simulink model "Controlador_codigo_export"  (R2023b)
settings: Solver=FixedStepAuto  StartTime=0.0  StopTime=20  FixedStep=0.00006  RelTol=1e-3
undefined symbols (not defined in the file): alpha_cu, b_eq, C_ts, g, J_eq, k_l, L_d, L_ls, L_q, lambda_m, magnitude, P_p, r, R_sREF, R_ts_amb, T_amb, T_ld, T_sdis, T_sREF, Tau_sens_temp, Vsat, w_n_modulador, w_n_sens_corr, w_n_sens_pos, zeta_mod, zeta_sens
libraries: SignalEditorBlockLib x2
settings Model: Creator=tomas  LastModifiedBy=tomas

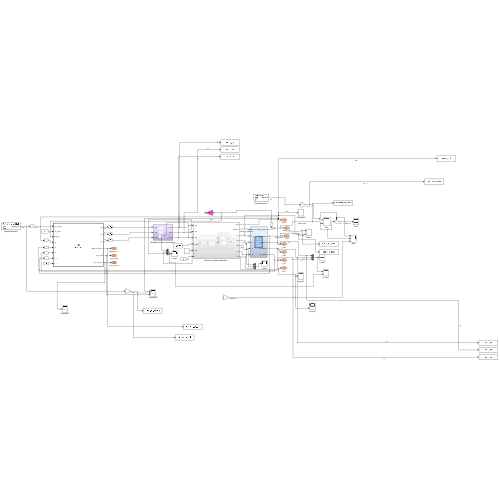
[thumbnail: Simulink's stored preview of the top-level diagram]
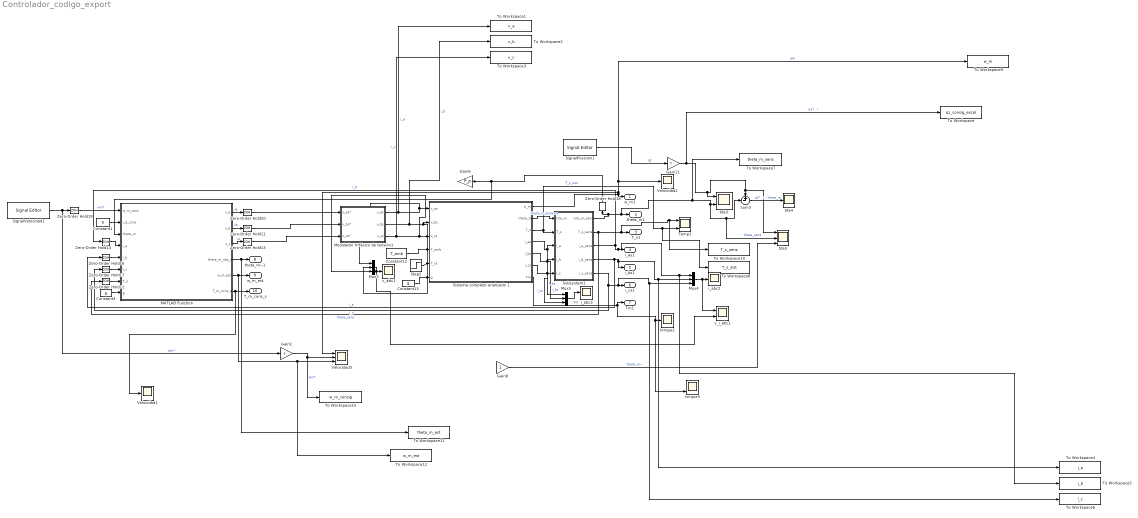
== system Controlador_codigo_export ==
  Constant1 : Constant  Value=0
  Constant12 : Constant  Value=T_amb
  Constant13 : Constant  Value=g
  Constant3 : Constant  Value=g
  Gain1 : Gain  Gain=r
  Gain11 : Gain  Gain=r
  Gain6 : Gain  Gain=P_p
  Gain8 : Gain
  MATLAB Function : MATLAB Function  TreatAsAtomicUnit=on
  Modulador trifásico de tensión1 : Subsystem
  Mux3 : Mux  Inputs=3
  Mux4 : Mux  Inputs=3
  Mux5 : Mux  Inputs=3
  SignalPosicion1 : SignalEditorBlockLib/Signal Editor  FileName=D:\Facu\Final AyME\Final-AyME\Simulink_LC\Simulacion\Signal\Perfil_trap_q1.mat  ActiveScenario=Scenarioq1  ActiveSignal=Signalq1  IsBus=off  OutputBusObjectStr=Bus: BusObject  SampleTime=0  ZeroCross=off  OutputAfterFinalValue=Holding final value  Unit=inherit  PreserveSignalName=on  ApplySigPropsToAllScenarios=on  ApplySigPropsToAllSignals=off
  SignalVelocidad1 : SignalEditorBlockLib/Signal Editor  FileName=D:\Facu\Final AyME\Final-AyME\Simulink_LC\Simulacion\Signal\Perfil_trap_velocidad.mat  ActiveScenario=Scenario_velocidad  ActiveSignal=Signal_vel  IsBus=off  OutputBusObjectStr=Bus: BusObject  SampleTime=0  ZeroCross=off  OutputAfterFinalValue=Holding final value  Unit=inherit  PreserveSignalName=on  ApplySigPropsToAllScenarios=on  ApplySigPropsToAllSignals=off
  Sistema completo analizado 1 : Subsystem
  Step2 : Step  Time=7.5  After=T_ld*0  SampleTime=0
  Subsystem1 : Subsystem
  Sum3 : Sum  Inputs=+-|
  Temp1 : Scope  NumInputPorts=2
  To Workspace : ToWorkspace  VariableName=q1_consig_escal  SaveFormat=Structure With Time  SampleTime=-1
  To Workspace1 : ToWorkspace  VariableName=v_a  SaveFormat=Structure With Time  SampleTime=-1
  To Workspace10 : ToWorkspace  VariableName=T_s_sens  SaveFormat=Structure With Time  SampleTime=-1
  To Workspace11 : ToWorkspace  VariableName=theta_m_est  SaveFormat=Structure With Time  SampleTime=-1
  To Workspace12 : ToWorkspace  VariableName=w_m_est  SaveFormat=Structure With Time  SampleTime=-1
  To Workspace15 : ToWorkspace  VariableName=w_m_consig  SaveFormat=Structure With Time  SampleTime=-1
  To Workspace2 : ToWorkspace  VariableName=v_b  SaveFormat=Structure With Time  SampleTime=-1
  To Workspace3 : ToWorkspace  VariableName=v_c  SaveFormat=Structure With Time  SampleTime=-1
  To Workspace4 : ToWorkspace  VariableName=i_a  SaveFormat=Structure With Time  SampleTime=-1
  To Workspace5 : ToWorkspace  VariableName=i_b  SaveFormat=Structure With Time  SampleTime=-1
  To Workspace6 : ToWorkspace  VariableName=i_c  SaveFormat=Structure With Time  SampleTime=-1
  To Workspace7 : ToWorkspace  VariableName=theta_m_sens  SaveFormat=Structure With Time  SampleTime=-1
  To Workspace8 : ToWorkspace  VariableName=T_s_sist  SaveFormat=Structure With Time  SampleTime=-1
  To Workspace9 : ToWorkspace  VariableName=w_m  SaveFormat=Structure With Time  SampleTime=-1
  Velocidad1 : Scope
  Velocidad2 : Scope
  Velocidad3 : Scope  NumInputPorts=3
  Zero-Order Hold{11..14,16..20} (9 alike) : ZeroOrderHold  SampleTime=T_sdis
  i_abc2 : Scope
  i_abc3 : Scope
  tita3 : Scope  NumInputPorts=2
  tita4 : Scope
  tita5 : Scope  NumInputPorts=3
  torque2 : Scope
  torque3 : Scope  NumInputPorts=2
  v_abc1 : Scope
  v_i_abc1 : Scope  NumInputPorts=2
  w_m1 : Outport
  theta_m1 : Outport  Port=2
  T_s1 : Outport  Port=3
  i_as1 : Outport  Port=4
  i_bs1 : Outport  Port=5
  i_cs1 : Outport  Port=6
  Tm1 : Outport  Port=7
  theta_m~1 : Outport  Port=8
  w_m_est : Outport  Port=9
  T_m_cons_s : Outport  Port=10
  wires:
  Sistema completo analizado 1/7(Tm) -> torque3/2, torque2/1, Tm1/1  "Tm"
  Zero-Order Hold11/1 -> Modulador trifásico de tensión1/2(v_bs*)
  Zero-Order Hold16/1 -> MATLAB Function/5(i_b)
  Zero-Order Hold18/1 -> MATLAB Function/3(theta_m), Gain6/1
  Step2/1 -> Sistema completo analizado 1/5(T_ld)
  MATLAB Function/2(v_b) -> Zero-Order Hold11/1  "vb"
  Sistema completo analizado 1/5(i_bs) -> Subsystem1/4(i_b), Mux5/2  "i_bs"
  Zero-Order Hold17/1 -> MATLAB Function/6(i_c)
  Zero-Order Hold13/1 -> Modulador trifásico de tensión1/3(v_cs*)
  Sistema completo analizado 1/2(theta_m) -> Subsystem1/1(tita_m)  "theta_m_sistema"
  Zero-Order Hold20/1 -> Modulador trifásico de tensión1/1(v_as*)
  Zero-Order Hold14/1 -> MATLAB Function/4(i_a)
  MATLAB Function/1(v_a) -> Zero-Order Hold20/1  "va"
  Mux4/1 -> v_i_abc1/1, i_abc2/1
  Constant1/1 -> MATLAB Function/2(i_d_cons)
  Mux5/1 -> i_abc3/1
  Sistema completo analizado 1/4(i_as) -> Subsystem1/3(i_a), Mux5/1  "i_as"
  Gain8/1 -> tita5/3  "theta_m~"
  Sum3/1 -> tita4/1  "q1* . r - theta_m"
  Constant3/1 -> MATLAB Function/8(g)
  Mux3/1 -> v_i_abc1/2, v_abc1/1
  Constant13/1 -> Sistema completo analizado 1/6(g)
  MATLAB Function/3(v_c) -> Zero-Order Hold13/1  "vc"
  Sistema completo analizado 1/3(T_s) -> Subsystem1/2(T_s), To Workspace8/1, Temp1/2  "T_s_sist"
  Sistema completo analizado 1/6(i_cs) -> Subsystem1/5(i_c), Mux5/3  "i_cs"
  Subsystem1/1(tita_m_sens) -> Zero-Order Hold18/1, To Workspace7/1, tita5/2, Sum3/2, tita3/2, theta_m1/1  "theta_sens"
  Constant12/1 -> Sistema completo analizado 1/4(T_amb)
  Zero-Order Hold12/1 -> MATLAB Function/7(T_s)
  MATLAB Function/6(T_m_cons_s) -> Velocidad1/1, T_m_cons_s/1
  Zero-Order Hold19/1 -> MATLAB Function/1(w_m_cons)  "wm*"
  SignalPosicion1/1 -> Gain11/1  "q1"
  Gain1/1 -> To Workspace15/1, Velocidad3/2  "wm*"
  Subsystem1/5(i_c_sens) -> Zero-Order Hold17/1, To Workspace6/1, Mux4/3, i_cs1/1  "i_c"
  Subsystem1/4(i_b_sens) -> i_bs1/1, To Workspace4/1, Mux4/2, Zero-Order Hold16/1  "i_a"
  Subsystem1/3(i_a_sens) -> To Workspace5/1, Mux4/1, i_as1/1, Zero-Order Hold14/1  "i_b"
  Subsystem1/2(T_s_sens) -> Zero-Order Hold12/1, To Workspace10/1, Temp1/1, T_s1/1  "theta_sens"
  Gain11/1 -> To Workspace/1, tita3/1, tita5/1, Sum3/1  "q1* . r"
  Sistema completo analizado 1/1(w_m) -> To Workspace9/1, Velocidad2/1, Velocidad3/1, w_m1/1  "wm"
  Modulador trifásico de tensión1/2(v_bs) -> To Workspace2/1, Mux3/2, Sistema completo analizado 1/2(v_bs)  "i_b"
  Modulador trifásico de tensión1/3(v_cs) -> To Workspace3/1, Mux3/3, Sistema completo analizado 1/3(v_cs)  "i_c"
  Modulador trifásico de tensión1/1(v_as) -> To Workspace1/1, Mux3/1, Sistema completo analizado 1/1(v_as)  "i_a"
  SignalVelocidad1/1 -> Gain1/1, Zero-Order Hold19/1  "wm*"
  MATLAB Function/5(w_m_est) -> To Workspace12/1, Velocidad3/3, w_m_est/1
  MATLAB Function/4(theta_m_obs_s) -> To Workspace11/1, theta_m~1/1

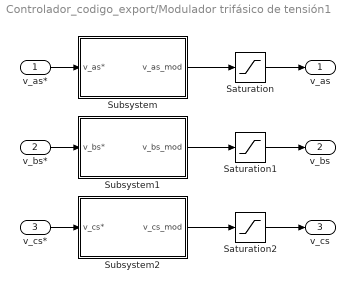
== system Controlador_codigo_export/Modulador trifásico de tensión1 ==
  v_as* : Inport
  v_bs* : Inport  Port=2
  v_cs* : Inport  Port=3
  Saturation : Saturate  UpperLimit=Vsat  LowerLimit=-Vsat
  Saturation1 : Saturate  UpperLimit=Vsat  LowerLimit=-Vsat
  Saturation2 : Saturate  UpperLimit=Vsat  LowerLimit=-Vsat
  Subsystem : Subsystem
  Subsystem1 : Subsystem
  Subsystem2 : Subsystem
  v_as : Outport
  v_bs : Outport  Port=2
  v_cs : Outport  Port=3
  wires:
  Subsystem/1(v_as_mod) -> Saturation/1
  Subsystem1/1(v_bs_mod) -> Saturation1/1
  Subsystem2/1(v_cs_mod) -> Saturation2/1
  v_cs*/1 -> Subsystem2/1(v_cs*)
  v_bs*/1 -> Subsystem1/1(v_bs*)
  v_as*/1 -> Subsystem/1(v_as*)
  Saturation/1 -> v_as/1
  Saturation1/1 -> v_bs/1
  Saturation2/1 -> v_cs/1

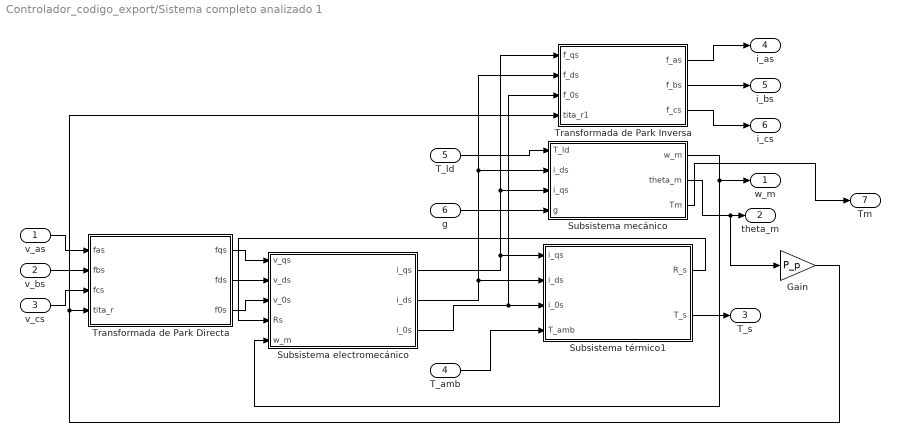
== system Controlador_codigo_export/Sistema completo analizado 1 ==
  v_as : Inport
  v_bs : Inport  Port=2
  v_cs : Inport  Port=3
  T_amb : Inport  Port=4
  T_ld : Inport  Port=5
  g : Inport  Port=6
  Gain : Gain  Gain=P_p
  Subsistema electromecánico : Subsystem
  Subsistema mecánico : Subsystem
  Subsistema térmico1 : Subsystem
  Transformada de Park Directa : Subsystem
  Transformada de Park Inversa : Subsystem
  w_m : Outport
  theta_m : Outport  Port=2
  T_s : Outport  Port=3
  i_as : Outport  Port=4
  i_bs : Outport  Port=5
  i_cs : Outport  Port=6
  Tm : Outport  Port=7
  wires:
  Transformada de Park Inversa/3(f_cs) -> i_cs/1
  Subsistema mecánico/1(w_m) -> w_m/1, Subsistema electromecánico/5(w_m)
  Subsistema electromecánico/3(i_0s) -> Subsistema térmico1/3(i_0s), Transformada de Park Inversa/3(f_0s)
  Transformada de Park Directa/1(fqs) -> Subsistema electromecánico/1(v_qs)
  Subsistema térmico1/2(T_s) -> T_s/1
  Transformada de Park Directa/3(f0s) -> Subsistema electromecánico/3(v_0s)
  Subsistema electromecánico/2(i_ds) -> Subsistema térmico1/2(i_ds), Transformada de Park Inversa/2(f_ds), Subsistema mecánico/2(i_ds)
  Gain/1 -> Transformada de Park Inversa/4(tita_r1), Transformada de Park Directa/4(tita_r)
  T_ld/1 -> Subsistema mecánico/1(T_ld)
  Transformada de Park Directa/2(fds) -> Subsistema electromecánico/2(v_ds)
  Transformada de Park Inversa/2(f_bs) -> i_bs/1
  v_bs/1 -> Transformada de Park Directa/2(fbs)
  T_amb/1 -> Subsistema térmico1/4(T_amb)
  Transformada de Park Inversa/1(f_as) -> i_as/1
  v_as/1 -> Transformada de Park Directa/1(fas)
  Subsistema mecánico/2(theta_m) -> Gain/1, theta_m/1
  v_cs/1 -> Transformada de Park Directa/3(fcs)
  Subsistema electromecánico/1(i_qs) -> Transformada de Park Inversa/1(f_qs), Subsistema mecánico/3(i_qs), Subsistema térmico1/1(i_qs)
  Subsistema térmico1/1(R_s) -> Subsistema electromecánico/4(Rs)
  g/1 -> Subsistema mecánico/4(g)
  Subsistema mecánico/3(Tm) -> Tm/1

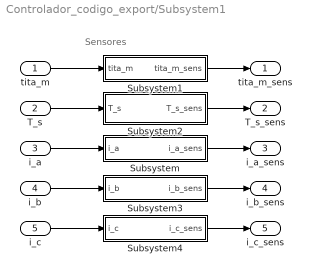
== system Controlador_codigo_export/Subsystem1 ==
  note: Sensores
  tita_m : Inport
  T_s : Inport  Port=2
  i_a : Inport  Port=3
  i_b : Inport  Port=4
  i_c : Inport  Port=5
  Subsystem : Subsystem
  Subsystem1 : Subsystem
  Subsystem2 : Subsystem
  Subsystem3 : Subsystem
  Subsystem4 : Subsystem
  tita_m_sens : Outport
  T_s_sens : Outport  Port=2
  i_a_sens : Outport  Port=3
  i_b_sens : Outport  Port=4
  i_c_sens : Outport  Port=5
  wires:
  tita_m/1 -> Subsystem1/1(tita_m)
  T_s/1 -> Subsystem2/1(T_s)
  i_a/1 -> Subsystem/1(i_a)
  i_b/1 -> Subsystem3/1(i_b)
  i_c/1 -> Subsystem4/1(i_c)
  Subsystem1/1(tita_m_sens) -> tita_m_sens/1
  Subsystem2/1(T_s_sens) -> T_s_sens/1
  Subsystem/1(i_a_sens) -> i_a_sens/1
  Subsystem3/1(i_b_sens) -> i_b_sens/1
  Subsystem4/1(i_c_sens) -> i_c_sens/1

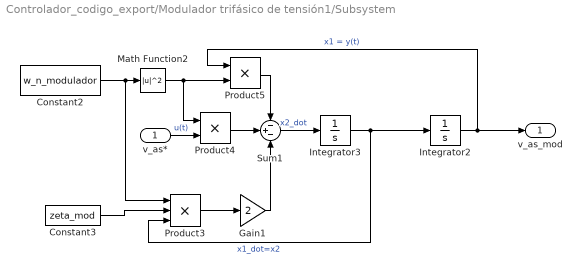
== system Controlador_codigo_export/Modulador trifásico de tensión1/Subsystem ==
  v_as* : Inport
  Constant2 : Constant  Value=w_n_modulador
  Constant3 : Constant  Value=zeta_mod
  Gain1 : Gain  Gain=2
  Integrator2 : Integrator
  Integrator3 : Integrator
  Math Function2 : Math  Operator=magnitude^2
  Product3 : Product  Inputs=3
  Product4 : Product
  Product5 : Product
  Sum1 : Sum  Inputs=-+-
  v_as_mod : Outport
  wires:
  Math Function2/1 -> Product5/2, Product4/1
  Integrator3/1 -> Product3/3, Integrator2/1  "x1_dot=x2"
  v_as*/1 -> Product4/2  "u(t)"
  Product4/1 -> Sum1/2
  Sum1/1 -> Integrator3/1  "x2_dot"
  Integrator2/1 -> v_as_mod/1, Product5/1  "x1 = y(t)"
  Gain1/1 -> Sum1/3
  Product3/1 -> Gain1/1
  Constant2/1 -> Product3/1, Math Function2/1
  Product5/1 -> Sum1/1
  Constant3/1 -> Product3/2

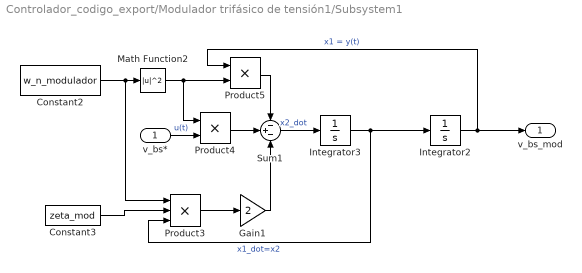
== system Controlador_codigo_export/Modulador trifásico de tensión1/Subsystem1 ==
  v_bs* : Inport
  Constant2 : Constant  Value=w_n_modulador
  Constant3 : Constant  Value=zeta_mod
  Gain1 : Gain  Gain=2
  Integrator2 : Integrator
  Integrator3 : Integrator
  Math Function2 : Math  Operator=magnitude^2
  Product3 : Product  Inputs=3
  Product4 : Product
  Product5 : Product
  Sum1 : Sum  Inputs=-+-
  v_bs_mod : Outport
  wires:
  Math Function2/1 -> Product5/2, Product4/1
  Integrator3/1 -> Product3/3, Integrator2/1  "x1_dot=x2"
  v_bs*/1 -> Product4/2  "u(t)"
  Product4/1 -> Sum1/2
  Sum1/1 -> Integrator3/1  "x2_dot"
  Integrator2/1 -> v_bs_mod/1, Product5/1  "x1 = y(t)"
  Gain1/1 -> Sum1/3
  Product3/1 -> Gain1/1
  Constant2/1 -> Product3/1, Math Function2/1
  Product5/1 -> Sum1/1
  Constant3/1 -> Product3/2

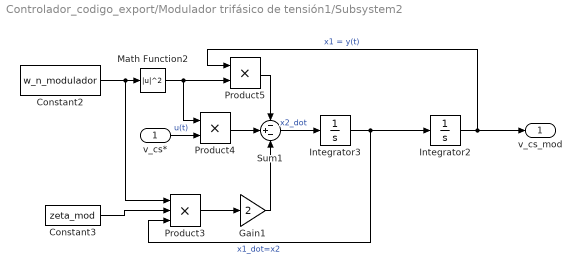
== system Controlador_codigo_export/Modulador trifásico de tensión1/Subsystem2 ==
  v_cs* : Inport
  Constant2 : Constant  Value=w_n_modulador
  Constant3 : Constant  Value=zeta_mod
  Gain1 : Gain  Gain=2
  Integrator2 : Integrator
  Integrator3 : Integrator
  Math Function2 : Math  Operator=magnitude^2
  Product3 : Product  Inputs=3
  Product4 : Product
  Product5 : Product
  Sum1 : Sum  Inputs=-+-
  v_cs_mod : Outport
  wires:
  Math Function2/1 -> Product5/2, Product4/1
  Integrator3/1 -> Product3/3, Integrator2/1  "x1_dot=x2"
  v_cs*/1 -> Product4/2  "u(t)"
  Product4/1 -> Sum1/2
  Sum1/1 -> Integrator3/1  "x2_dot"
  Integrator2/1 -> v_cs_mod/1, Product5/1  "x1 = y(t)"
  Gain1/1 -> Sum1/3
  Product3/1 -> Gain1/1
  Constant2/1 -> Product3/1, Math Function2/1
  Product5/1 -> Sum1/1
  Constant3/1 -> Product3/2

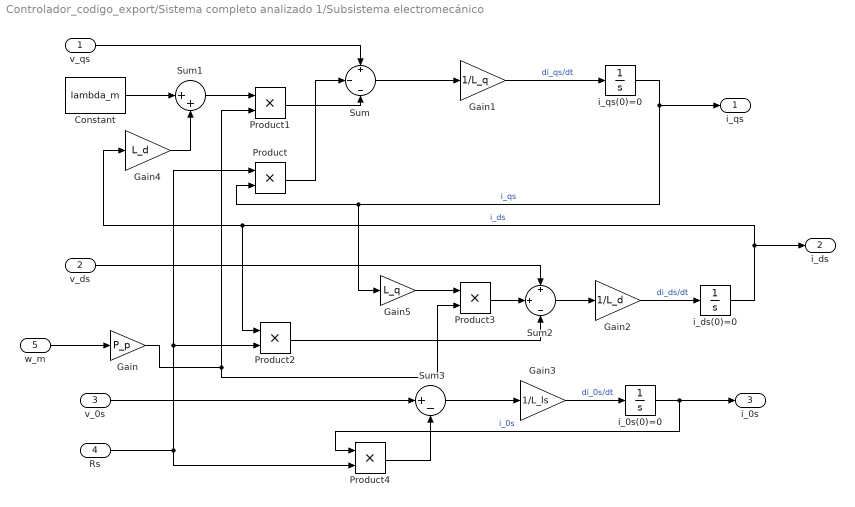
== system Controlador_codigo_export/Sistema completo analizado 1/Subsistema electromecánico ==
  v_qs : Inport
  v_ds : Inport  Port=2
  v_0s : Inport  Port=3
  Rs : Inport  Port=4
  w_m : Inport  Port=5
  Constant : Constant  Value=lambda_m
  Gain : Gain  Gain=P_p
  Gain1 : Gain  Gain=1/L_q
  Gain2 : Gain  Gain=1/L_d
  Gain3 : Gain  Gain=1/L_ls
  Gain4 : Gain  Gain=L_d
  Gain5 : Gain  Gain=L_q
  Product{,1..4} (5 alike) : Product
  Sum : Sum  Inputs=+|-|-
  Sum1 : Sum  Inputs=|++
  Sum2 : Sum  Inputs=+|+|-
  Sum3 : Sum  Inputs=|+-
  i_0s(0)=0 : Integrator
  i_ds(0)=0 : Integrator
  i_qs(0)=0 : Integrator
  i_qs : Outport
  i_ds : Outport  Port=2
  i_0s : Outport  Port=3
  wires:
  Gain1/1 -> i_qs(0)=0/1  "di_qs/dt"
  Rs/1 -> Product2/2, Product/1, Product4/2
  i_qs(0)=0/1 -> Gain5/1, Product/2, i_qs/1  "i_qs"
  Sum2/1 -> Gain2/1
  Product1/1 -> Sum/3
  Product4/1 -> Sum3/2
  v_0s/1 -> Sum3/1
  Product3/1 -> Sum2/2
  Gain3/1 -> i_0s(0)=0/1  "di_0s/dt"
  Gain/1 -> Product3/2, Product1/2
  v_qs/1 -> Sum/1
  Sum1/1 -> Product1/1
  Gain5/1 -> Product3/1
  Sum3/1 -> Gain3/1
  i_0s(0)=0/1 -> Product4/1, i_0s/1  "i_0s"
  Product2/1 -> Sum2/3
  Gain2/1 -> i_ds(0)=0/1  "di_ds/dt"
  Constant/1 -> Sum1/1
  Gain4/1 -> Sum1/2
  Sum/1 -> Gain1/1
  Product/1 -> Sum/2
  w_m/1 -> Gain/1
  i_ds(0)=0/1 -> Product2/1, Gain4/1, i_ds/1  "i_ds"
  v_ds/1 -> Sum2/1

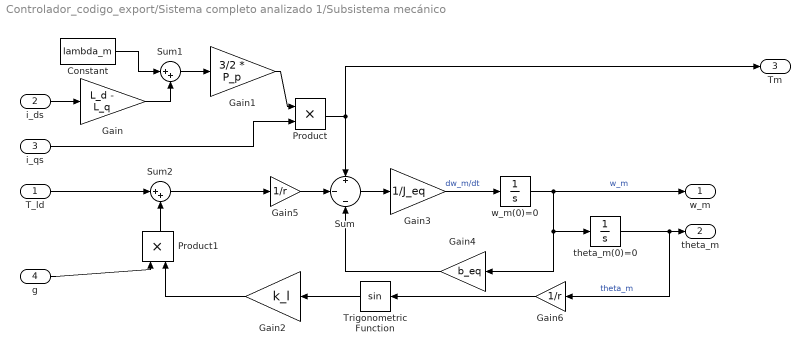
== system Controlador_codigo_export/Sistema completo analizado 1/Subsistema mecánico ==
  T_ld : Inport
  i_ds : Inport  Port=2
  i_qs : Inport  Port=3
  g : Inport  Port=4
  Constant : Constant  Value=lambda_m
  Gain : Gain  Gain=L_d - L_q
  Gain1 : Gain  Gain=3/2 * P_p
  Gain2 : Gain  Gain=k_l
  Gain3 : Gain  Gain=1/J_eq
  Gain4 : Gain  Gain=b_eq
  Gain5 : Gain  Gain=1/r
  Gain6 : Gain  Gain=1/r
  Product : Product
  Product1 : Product
  Sum : Sum  Inputs=+|-|-
  Sum1 : Sum  Inputs=|++
  Sum2 : Sum  Inputs=|++
  Trigonometric Function : Trigonometry
  theta_m(0)=0 : Integrator
  w_m(0)=0 : Integrator
  w_m : Outport
  theta_m : Outport  Port=2
  Tm : Outport  Port=3
  wires:
  w_m(0)=0/1 -> w_m/1, theta_m(0)=0/1, Gain4/1  "w_m"
  Sum/1 -> Gain3/1
  Gain3/1 -> w_m(0)=0/1  "dw_m/dt"
  i_ds/1 -> Gain/1
  Constant/1 -> Sum1/1
  Gain/1 -> Sum1/2
  Sum1/1 -> Gain1/1
  Gain1/1 -> Product/1
  i_qs/1 -> Product/2
  Gain4/1 -> Sum/3
  Gain5/1 -> Sum/2
  Trigonometric Function/1 -> Gain2/1
  Gain2/1 -> Product1/2
  theta_m(0)=0/1 -> Gain6/1, theta_m/1  "theta_m"
  T_ld/1 -> Sum2/1
  Sum2/1 -> Gain5/1
  Gain6/1 -> Trigonometric Function/1
  g/1 -> Product1/1
  Product1/1 -> Sum2/2
  Product/1 -> Sum/1, Tm/1

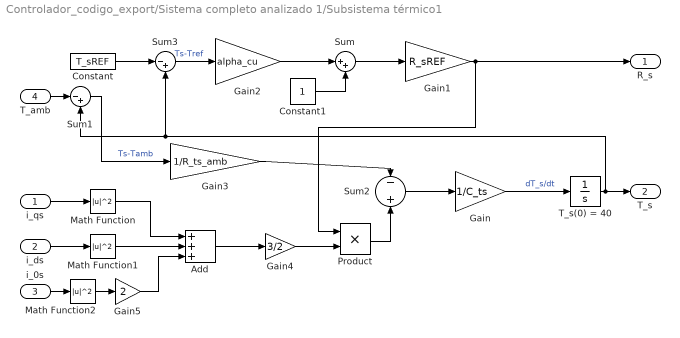
== system Controlador_codigo_export/Sistema completo analizado 1/Subsistema térmico1 ==
  i_qs : Inport
  i_ds : Inport  Port=2
  i_0s : Inport  Port=3
  T_amb : Inport  Port=4
  Add : Sum  Inputs=+++
  Constant : Constant  Value=T_sREF
  Constant1 : Constant
  Gain : Gain  Gain=1/C_ts
  Gain1 : Gain  Gain=R_sREF
  Gain2 : Gain  Gain=alpha_cu
  Gain3 : Gain  Gain=1/R_ts_amb
  Gain4 : Gain  Gain=3/2
  Gain5 : Gain  Gain=2
  Math Function : Math  Operator=magnitude^2
  Math Function1 : Math  Operator=magnitude^2
  Math Function2 : Math  Operator=magnitude^2
  Product : Product
  Sum : Sum  Inputs=|++
  Sum1 : Sum  Inputs=|-+
  Sum2 : Sum  Inputs=-|+
  Sum3 : Sum  Inputs=|-+
  T_s(0) = 40 : Integrator  InitialCondition=40
  R_s : Outport
  T_s : Outport  Port=2
  wires:
  Math Function2/1 -> Gain5/1
  Math Function/1 -> Add/1
  T_amb/1 -> Sum1/1
  Sum2/1 -> Gain/1
  Sum/1 -> Gain1/1
  Gain2/1 -> Sum/1
  Gain1/1 -> Product/1, R_s/1
  i_ds/1 -> Math Function1/1
  Gain/1 -> T_s(0) = 40/1  "dT_s/dt"
  Constant1/1 -> Sum/2
  Gain4/1 -> Product/2
  T_s(0) = 40/1 -> T_s/1, Sum3/2, Sum1/2
  Math Function1/1 -> Add/2
  i_0s/1 -> Math Function2/1
  Sum1/1 -> Gain3/1  "Ts-Tamb"
  Add/1 -> Gain4/1
  Gain5/1 -> Add/3
  i_qs/1 -> Math Function/1
  Gain3/1 -> Sum2/1
  Product/1 -> Sum2/2
  Constant/1 -> Sum3/1
  Sum3/1 -> Gain2/1  "Ts-Tref"

== system Controlador_codigo_export/Sistema completo analizado 1/Transformada de Park Directa ==
  fas : Inport
  fbs : Inport  Port=2
  fcs : Inport  Port=3
  tita_r : Inport  Port=4
  MATLAB Function1 : MATLAB Function  TreatAsAtomicUnit=on
  fqs : Outport
  fds : Outport  Port=2
  f0s : Outport  Port=3
  wires:
  fas/1 -> MATLAB Function1/1(f_as)
  MATLAB Function1/3(f_0s) -> f0s/1
  MATLAB Function1/2(f_ds) -> fds/1
  fbs/1 -> MATLAB Function1/2(f_bs)
  fcs/1 -> MATLAB Function1/3(f_cs)
  tita_r/1 -> MATLAB Function1/4(tita_r)
  MATLAB Function1/1(f_qs) -> fqs/1

== system Controlador_codigo_export/Sistema completo analizado 1/Transformada de Park Inversa ==
  f_qs : Inport
  f_ds : Inport  Port=2
  f_0s : Inport  Port=3
  tita_r1 : Inport  Port=4
  MATLAB Function2 : MATLAB Function  TreatAsAtomicUnit=on
  f_as : Outport
  f_bs : Outport  Port=2
  f_cs : Outport  Port=3
  wires:
  tita_r1/1 -> MATLAB Function2/4(tita_r)
  MATLAB Function2/2(f_bs) -> f_bs/1
  MATLAB Function2/1(f_as) -> f_as/1
  f_ds/1 -> MATLAB Function2/2(f_ds)
  MATLAB Function2/3(f_cs) -> f_cs/1
  f_0s/1 -> MATLAB Function2/3(f_0s)
  f_qs/1 -> MATLAB Function2/1(f_qs)

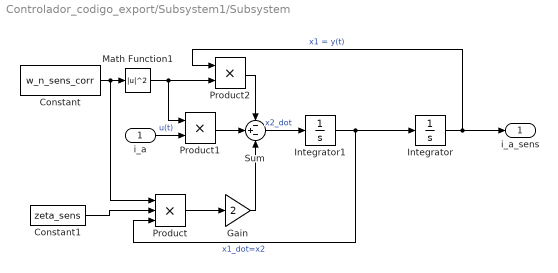
== system Controlador_codigo_export/Subsystem1/Subsystem ==
  i_a : Inport
  Constant : Constant  Value=w_n_sens_corr
  Constant1 : Constant  Value=zeta_sens
  Gain : Gain  Gain=2
  Integrator : Integrator
  Integrator1 : Integrator
  Math Function1 : Math  Operator=magnitude^2
  Product : Product  Inputs=3
  Product1 : Product
  Product2 : Product
  Sum : Sum  Inputs=-+-
  i_a_sens : Outport
  wires:
  Product1/1 -> Sum/2
  Gain/1 -> Sum/3
  Constant/1 -> Product/1, Math Function1/1
  i_a/1 -> Product1/2  "u(t)"
  Product/1 -> Gain/1
  Product2/1 -> Sum/1
  Math Function1/1 -> Product2/2, Product1/1
  Sum/1 -> Integrator1/1  "x2_dot"
  Constant1/1 -> Product/2
  Integrator1/1 -> Product/3, Integrator/1  "x1_dot=x2"
  Integrator/1 -> i_a_sens/1, Product2/1  "x1 = y(t)"

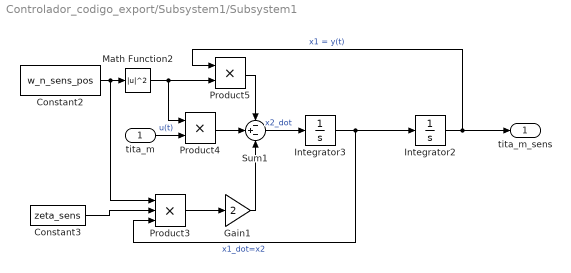
== system Controlador_codigo_export/Subsystem1/Subsystem1 ==
  tita_m : Inport
  Constant2 : Constant  Value=w_n_sens_pos
  Constant3 : Constant  Value=zeta_sens
  Gain1 : Gain  Gain=2
  Integrator2 : Integrator
  Integrator3 : Integrator
  Math Function2 : Math  Operator=magnitude^2
  Product3 : Product  Inputs=3
  Product4 : Product
  Product5 : Product
  Sum1 : Sum  Inputs=-+-
  tita_m_sens : Outport
  wires:
  Constant2/1 -> Product3/1, Math Function2/1
  Gain1/1 -> Sum1/3
  Product4/1 -> Sum1/2
  Integrator3/1 -> Product3/3, Integrator2/1  "x1_dot=x2"
  Product3/1 -> Gain1/1
  Constant3/1 -> Product3/2
  Math Function2/1 -> Product5/2, Product4/1
  Product5/1 -> Sum1/1
  tita_m/1 -> Product4/2  "u(t)"
  Sum1/1 -> Integrator3/1  "x2_dot"
  Integrator2/1 -> tita_m_sens/1, Product5/1  "x1 = y(t)"

== system Controlador_codigo_export/Subsystem1/Subsystem2 ==
  T_s : Inport
  Constant4 : Constant  Value=1/Tau_sens_temp
  Integrator4 : Integrator  InitialCondition=40
  Product6 : Product
  Sum2 : Sum  Inputs=|+-
  T_s_sens : Outport
  wires:
  T_s/1 -> Sum2/1  "u(t)"
  Product6/1 -> Integrator4/1  "x_dot"
  Constant4/1 -> Product6/1
  Integrator4/1 -> Sum2/2, T_s_sens/1  "x = y(t)"
  Sum2/1 -> Product6/2

== system Controlador_codigo_export/Subsystem1/Subsystem3 ==
  i_b : Inport
  Constant : Constant  Value=w_n_sens_corr
  Constant1 : Constant  Value=zeta_sens
  Gain : Gain  Gain=2
  Integrator : Integrator
  Integrator1 : Integrator
  Math Function1 : Math  Operator=magnitude^2
  Product : Product  Inputs=3
  Product1 : Product
  Product2 : Product
  Sum : Sum  Inputs=-+-
  i_b_sens : Outport
  wires:
  Product1/1 -> Sum/2
  Gain/1 -> Sum/3
  Constant/1 -> Product/1, Math Function1/1
  i_b/1 -> Product1/2  "u(t)"
  Product/1 -> Gain/1
  Product2/1 -> Sum/1
  Math Function1/1 -> Product2/2, Product1/1
  Sum/1 -> Integrator1/1  "x2_dot"
  Constant1/1 -> Product/2
  Integrator1/1 -> Product/3, Integrator/1  "x1_dot=x2"
  Integrator/1 -> i_b_sens/1, Product2/1  "x1 = y(t)"

== system Controlador_codigo_export/Subsystem1/Subsystem4 ==
  i_c : Inport
  Constant : Constant  Value=w_n_sens_corr
  Constant1 : Constant  Value=zeta_sens
  Gain : Gain  Gain=2
  Integrator : Integrator
  Integrator1 : Integrator
  Math Function1 : Math  Operator=magnitude^2
  Product : Product  Inputs=3
  Product1 : Product
  Product2 : Product
  Sum : Sum  Inputs=-+-
  i_c_sens : Outport
  wires:
  Product1/1 -> Sum/2
  Gain/1 -> Sum/3
  Constant/1 -> Product/1, Math Function1/1
  i_c/1 -> Product1/2  "u(t)"
  Product/1 -> Gain/1
  Product2/1 -> Sum/1
  Math Function1/1 -> Product2/2, Product1/1
  Sum/1 -> Integrator1/1  "x2_dot"
  Constant1/1 -> Product/2
  Integrator1/1 -> Product/3, Integrator/1  "x1_dot=x2"
  Integrator/1 -> i_c_sens/1, Product2/1  "x1 = y(t)"

== matlab function Controlador_codigo_export/MATLAB Function ==
  data: w_m_cons input; v_a output; i_d_cons input; theta_m input; i_a input; i_b input; i_c input; T_s input; g input; v_b output; v_c output; theta_m_obs_s output; w_m_est output; T_m_cons_s output
function [v_a,v_b,v_c,theta_m_obs_s,w_m_est,T_m_cons_s]=Controlador(w_m_cons,i_d_cons,theta_m,i_a,i_b,i_c,T_s,g)    
    %%Variables auxiliares
    P_p=3;
    T_sREF = 20;
    alpha_cu=3.9*10^-3;
    R_sREF=1.02;
    J_nom=1.9785e-5;

    theta_r=theta_m*P_p;
    

    %Variables Observador
    K_obs_theta=6400;   
    K_obs_w=10240000;
    persistent theta_m_obs;
    persistent w_m_obs_ant;
    persistent dw_m_obs_ant;
    persistent theta_m_obs_ant;
    persistent dtheta_m_obs_ant;

    %Variables PID

    w_n_PID=800;
    zeta_PID=0.75;

    b_a=J_nom*(2*zeta_PID+1)*w_n_PID;
    K_a=J_nom*(2*zeta_PID+1)*w_n_PID^2;
    K_ai=J_nom*w_n_PID^3;
    
    persistent T_m_cons;
    persistent theta_m_cons_ant;
    persistent w_m_cons_ant;
    persistent int_e_theta_m_PID_ant;
    persistent e_theta_m_PID_ant;


    %Variables persistentes
    persistent init;
    
    
   if isempty(init)
        init = true;
        
        theta_m_obs=0;
        w_m_obs_ant=0;
        dw_m_obs_ant=0;
        theta_m_obs_ant=0;
        dtheta_m_obs_ant=0;

        T_m_cons=0;
        theta_m_cons_ant=0;
        w_m_cons_ant=0;
        int_e_theta_m_PID_ant=0;
        e_theta_m_PID_ant=0;
   end
    %%
    %%Estimacion de resistencia
    R_s=R_sREF*(1+alpha_cu*(T_s-T_sREF));
    
    %%
    %%Transformada de park directa
    i_qd0 = 2/3 * [cos(theta_r), cos(theta_r - 2*pi/3), cos(theta_r + 2*pi/3);
                    sin(theta_r), sin(theta_r - 2*pi/3), sin(theta_r + 2*pi/3);
                    1/2, 1/2, 1/2] * [i_a;i_b;i_c];
    i_q=i_qd0(1);
    i_d=i_qd0(2);
    i_0=i_qd0(3);
    
    %%
    %%Observador
    e_theta_m_obs=theta_m-theta_m_obs;
    dw_m_obs=K_obs_w*e_theta_m_obs+T_m_cons/J_nom;
    [w_m_obs,w_m_obs_ant,dw_m_obs_ant]=integralTustin(dw_m_obs,w_m_obs_ant,dw_m_obs_ant);
    dtheta_m_obs=w_m_obs+K_obs_theta*e_theta_m_obs;
    [theta_m_obs,theta_m_obs_ant,dtheta_m_obs_ant]=integralTustin(dtheta_m_obs,theta_m_obs_ant,dtheta_m_obs_ant);
    w_m_est=dtheta_m_obs;
   
    %%
    %%PID
    r = 120/1;
    w_m_cons_escalado = w_m_cons * r;
    e_w_m_PID=w_m_cons_escalado-w_m_est;
    [theta_m_cons,theta_m_cons_ant,w_m_cons_ant]=integralTustin(w_m_cons_escalado,theta_m_cons_ant,w_m_cons_ant);
    e_theta_m_PID=theta_m_cons-theta_m;
    [int_e_theta_m_PID,int_e_theta_m_PID_ant,e_theta_m_PID_ant]=integralTustin(e_theta_m_PID,int_e_theta_m_PID_ant,e_theta_m_PID_ant);
    T_m_cons=b_a*e_w_m_PID+K_a*e_theta_m_PID+K_ai*int_e_theta_m_PID;
   
    %%
    %%MODULADOR DE TORQUE
    %Desacople de tensiones
    m = 1;
    L_cm = 0.25;
    m_l_nom = 0;
    b_l_nom =0.1;
    L_l = 0.5; 
    b_m = 15.0*10^-6;
    b_nom = b_m + b_l_nom/(r^2);
    k_l_nom = m * L_cm + m_l_nom * L_l;
    L_d = 6.6 * 10^(-3);
    L_q=5.8 * 10^(-3);
    L_ls = 0.8 * 10^(-3);
    lambda_m = 0.016;
    R_q=29;
    R_d=33;
    R_0=4;
    i_q_cons=(T_m_cons+b_nom*w_m_est+(k_l_nom*g)/(r)*sin(theta_m/r))/(3*P_p/2*((L_d-L_q)*i_d+lambda_m));
    i_0_cons = 0;

    %Lazos de corriente
    v_q_cons=R_q*(i_q_cons-i_q);
    v_d_cons=R_d*(i_d_cons-i_d);
    v_0_cons=R_0*(i_0_cons-i_0);

    v_q=v_q_cons+R_s*i_q+(lambda_m+L_d*i_d)*P_p*w_m_est;
    v_d=v_d_cons+R_s*i_d-L_q*i_q*P_p*w_m_est;
    v_0=v_0_cons+R_s*i_0;

    %%Transformada de park inversa
    v_abc = [cos(theta_r), sin(theta_r), 1;
             cos(theta_r - 2*pi/3), sin(theta_r - 2*pi/3), 1;
             cos(theta_r + 2*pi/3), sin(theta_r + 2*pi/3), 1] * [v_q;v_d;v_0];
    v_a=v_abc(1);
    v_b=v_abc(2);
    v_c=v_abc(3);

    %Salidas persistentes
    theta_m_obs_s=theta_m_obs;
    T_m_cons_s=T_m_cons;
end

function [y,y_ant,x_ant]=integralTustin(x,y_ant,x_ant)
    T_sdis = 6*10^-5; 
    y=y_ant+T_sdis/2 * (x+x_ant);
    y_ant=y;
    x_ant=x;
end

== matlab function Controlador_codigo_export/Sistema completo analizado 1/Transformada de Park Directa/MATLAB Function1 ==
  data: f_as input; f_qs output; f_bs input; f_cs input; tita_r input; f_ds output; f_0s output
function [f_qs, f_ds, f_0s] = parkDir(f_as,f_bs,f_cs,tita_r)

answer = 2/3 * [cos(tita_r), cos(tita_r - 2*pi/3), cos(tita_r + 2*pi/3);
         sin(tita_r), sin(tita_r - 2*pi/3), sin(tita_r + 2*pi/3);
         1/2, 1/2, 1/2] * [f_as;f_bs;f_cs];

f_qs = answer(1);
f_ds = answer(2);
f_0s = answer(3);

== matlab function Controlador_codigo_export/Sistema completo analizado 1/Transformada de Park Inversa/MATLAB Function2 ==
  data: f_qs input; f_as output; f_ds input; f_0s input; tita_r input; f_bs output; f_cs output
function [f_as, f_bs, f_cs] = parkInv(f_qs,f_ds,f_0s,tita_r)

answer = [cos(tita_r), sin(tita_r), 1;
         cos(tita_r - 2*pi/3), sin(tita_r - 2*pi/3), 1;
         cos(tita_r + 2*pi/3), sin(tita_r + 2*pi/3), 1] * [f_qs;f_ds;f_0s]; 

f_as = answer(1);
f_bs = answer(2);
f_cs = answer(3);
